simulink model "ex_4"  (R2023b)
settings: Solver=VariableStepAuto  StartTime=0.0  StopTime=10  RelTol=1e-3
values from neighbouring files (symbols this model uses):
  K_1 = 7    [ex_5.m]
  K_2 = 7    [ex_5.m]
undefined symbols (not defined in the file or in its folder): b, t_f, x_f, y_1_dot_end, y_1_end, y_2_dot_end, y_2_end, y_f
libraries: robotmobilelib x1
settings Model: Creator=savio  LastModifiedBy=savio

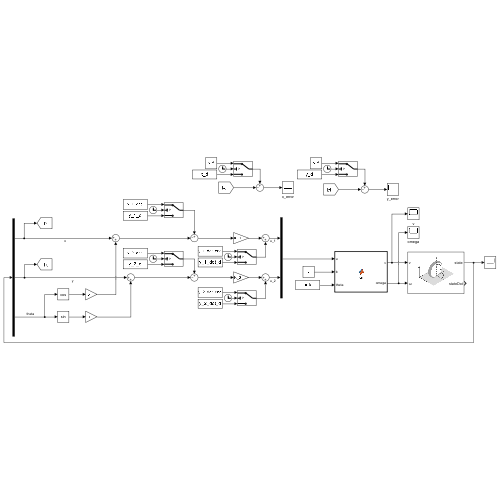
[thumbnail: Simulink's stored preview of the top-level diagram]
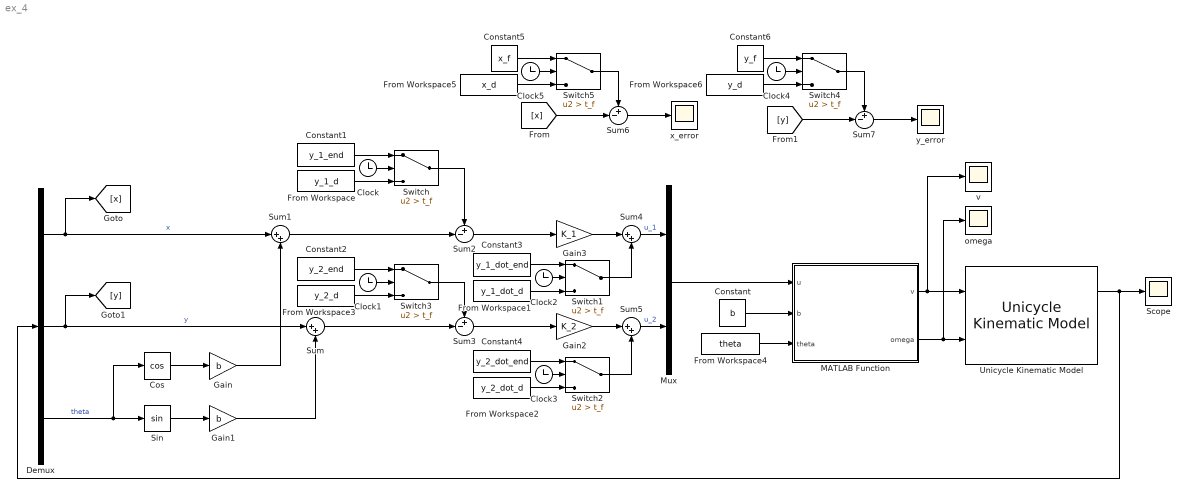
== system ex_4 ==
  Clock{,1..5} (6 alike) : Clock
  Constant : Constant  Value=b
  Constant1 : Constant  Value=y_1_end
  Constant2 : Constant  Value=y_2_end
  Constant3 : Constant  Value=y_1_dot_end
  Constant4 : Constant  Value=y_2_dot_end
  Constant5 : Constant  Value=x_f
  Constant6 : Constant  Value=y_f
  Cos : Trigonometry  Operator=cos
  Demux : Demux  Outputs=3
  From Workspace : FromWorkspace  VariableName=y_1_d
  From Workspace1 : FromWorkspace  VariableName=y_1_dot_d
  From Workspace2 : FromWorkspace  VariableName=y_2_dot_d
  From Workspace3 : FromWorkspace  VariableName=y_2_d
  From Workspace4 : FromWorkspace  VariableName=theta
  From Workspace5 : FromWorkspace  VariableName=x_d
  From Workspace6 : FromWorkspace  VariableName=y_d
  Gain : Gain  Gain=b
  Gain1 : Gain  Gain=b
  Gain2 : Gain  Gain=K_2
  Gain3 : Gain  Gain=K_1
  MATLAB Function : MATLAB Function  TreatAsAtomicUnit=on
  Mux : Mux  Inputs=2
  Scope : Scope
  Sin : Trigonometry
  Sum{,1,4..5} (4 alike) : Sum  Inputs=|++
  Sum{2..3,6..7} (4 alike) : Sum  Inputs=+-|
  Switch{,1..5} (6 alike) : Switch  Criteria=u2 > Threshold  Threshold=t_f  SaturateOnIntegerOverflow=off  InputSameDT=off
  Unicycle Kinematic Model : robotmobilelib/Unicycle Kinematic Model  VehicleInputs=Vehicle Speed & Heading Angular Velocity  WheelRadius=0.1  WheelSpeedRange=[-Inf Inf]  InitialState=[0; 0; 0]  SimulateUsing=Interpreted execution
  omega : Scope
  v : Scope
  x_error : Scope
  y_error : Scope
  wires:
  Unicycle Kinematic Model/1 -> Scope/1, Demux/1
  Demux/3 -> Cos/1, Sin/1  "theta"
  Demux/1 -> [x], Sum1/1  "x"
  Cos/1 -> Gain/1
  Sin/1 -> Gain1/1
  Demux/2 -> [y], Sum/1  "y"
  Gain/1 -> Sum1/2
  Gain1/1 -> Sum/2
  Sum1/1 -> Sum2/2
  Sum/1 -> Sum3/2
  Sum3/1 -> Gain2/1
  Sum2/1 -> Gain3/1
  Gain3/1 -> Sum4/1
  Gain2/1 -> Sum5/1
  Sum5/1 -> Mux/2  "u_2"
  Sum4/1 -> Mux/1  "u_1"
  Mux/1 -> MATLAB Function/1(u)
  Constant/1 -> MATLAB Function/2(b)
  From Workspace4/1 -> MATLAB Function/3(theta)
  MATLAB Function/1(v) -> v/1, Unicycle Kinematic Model/1
  MATLAB Function/2(omega) -> omega/1, Unicycle Kinematic Model/2
  [x] -> Sum6/2
  [y] -> Sum7/2
  Sum6/1 -> x_error/1
  Sum7/1 -> y_error/1
  Switch/1 -> Sum2/1
  Clock/1 -> Switch/2
  Switch3/1 -> Sum3/1
  Clock1/1 -> Switch3/2
  Clock2/1 -> Switch1/2
  Switch2/1 -> Sum5/2
  Clock3/1 -> Switch2/2
  Constant1/1 -> Switch/1
  From Workspace/1 -> Switch/3
  From Workspace3/1 -> Switch3/3
  Constant2/1 -> Switch3/1
  Constant3/1 -> Switch1/1
  From Workspace1/1 -> Switch1/3
  Constant4/1 -> Switch2/1
  From Workspace2/1 -> Switch2/3
  Switch1/1 -> Sum4/2
  Constant6/1 -> Switch4/1
  Clock4/1 -> Switch4/2
  From Workspace6/1 -> Switch4/3
  Constant5/1 -> Switch5/1
  From Workspace5/1 -> Switch5/3
  Clock5/1 -> Switch5/2
  Switch5/1 -> Sum6/1
  Switch4/1 -> Sum7/1

== matlab function ex_4/MATLAB Function ==
  data: u input; v output; b input; theta input; omega output
function [v, omega] = fcn(u, b, theta)

T = [cos(theta)  -b*sin(theta)
     sin(theta)   b*cos(theta)];

y = inv(T)*u;
v = y(1);
omega = y(2);
